simulink model "six_dof_COMPUTED_TORQUE"  (R2021b)
settings: Solver=ode4  StartTime=0.0  StopTime=10.0  FixedStep=1/100  RelTol=1e-3
libraries: robotmaniplib x4, simulink x2
settings Model: Creator=HP  LastModifiedBy=marco

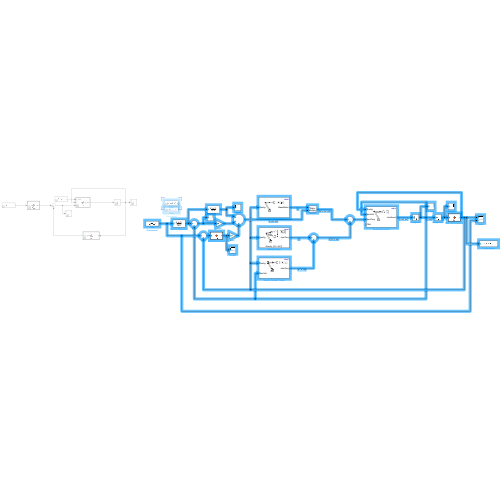
[thumbnail: Simulink's stored preview of the top-level diagram]
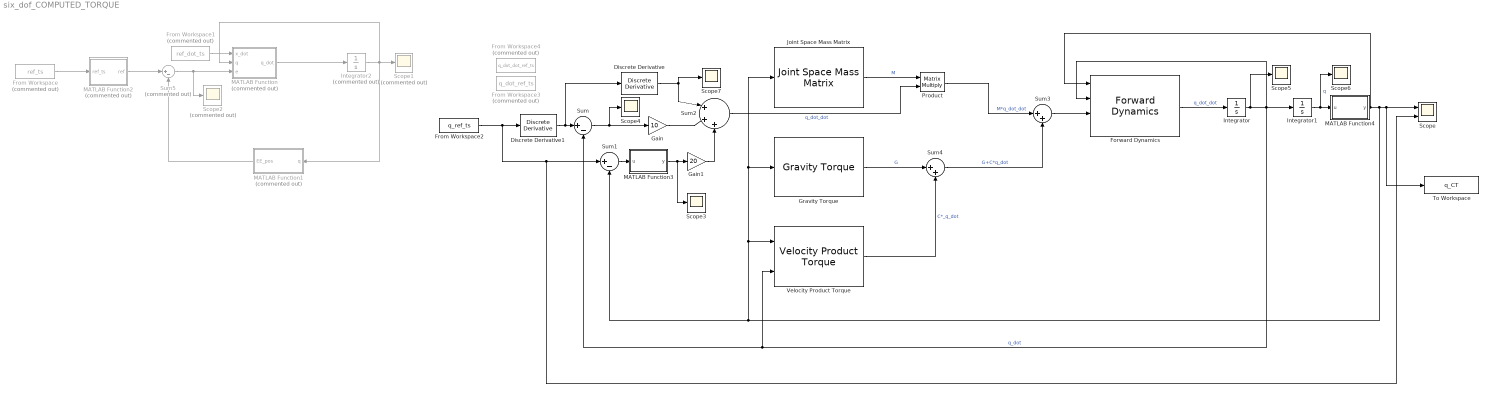
== system six_dof_COMPUTED_TORQUE ==
  Discrete Derivative : simulink/Discrete/Discrete Derivative  gainval=1.0  ICPrevScaledInput=0.0  OutMin=[]  OutMax=[]  OutDataType=fixdt(1, 16)  OutScaling=2^-10  DoSatur=off
  Discrete Derivative1 : simulink/Discrete/Discrete Derivative  gainval=1.0  ICPrevScaledInput=0.0  OutMin=[]  OutMax=[]  OutDataType=fixdt(1, 16)  OutScaling=2^-10  DoSatur=off
  Forward Dynamics : robotmaniplib/Forward Dynamics  RigidBodyTree=robot  SimulateUsing=Interpreted execution
  From Workspace : FromWorkspace  Commented=on  VariableName=ref_ts
  From Workspace1 : FromWorkspace  Commented=on  VariableName=ref_dot_ts
  From Workspace2 : FromWorkspace  VariableName=q_ref_ts
  From Workspace3 : FromWorkspace  Commented=on  VariableName=q_dot_ref_ts
  From Workspace4 : FromWorkspace  Commented=on  VariableName=q_dot_dot_ref_ts
  Gain : Gain  Gain=10
  Gain1 : Gain  Gain=20
  Gravity Torque : robotmaniplib/Gravity Torque  RigidBodyTree=robot  SimulateUsing=Interpreted execution
  Integrator : Integrator  InitialCondition=[0; 0; 0; 0; 0; 0]  LimitOutput=on  UpperSaturationLimit=[pi/2; pi/2; pi/2; pi/2; pi/2; pi/2]  LowerSaturationLimit=-[pi/2; pi/2; pi/2; pi/2; pi/2; pi/2]
  Integrator1 : Integrator  InitialCondition=[0; 0; 0; 0; pi/2; 0]  LimitOutput=on  UpperSaturationLimit=[pi; pi/4; 5*pi/4; pi; 5*pi/4; pi]  LowerSaturationLimit=-[pi; 5*pi/4; pi/4; pi; 5*pi/4; pi]
  Integrator2 : Integrator  Commented=on
  Joint Space Mass Matrix : robotmaniplib/Joint Space Mass Matrix  RigidBodyTree=robot  SimulateUsing=Interpreted execution
  MATLAB Function : MATLAB Function  Commented=on  TreatAsAtomicUnit=on
  MATLAB Function1 : MATLAB Function  Commented=on  TreatAsAtomicUnit=on
  MATLAB Function2 : MATLAB Function  Commented=on  TreatAsAtomicUnit=on
  MATLAB Function3 : MATLAB Function  TreatAsAtomicUnit=on
  MATLAB Function4 : MATLAB Function  TreatAsAtomicUnit=on
  Product : Product  Multiplication=Matrix(*)
  Scope : Scope  NumInputPorts=2
  Scope1 : Scope  Commented=on
  Scope2 : Scope  Commented=on
  Scope{3..7} (5 alike) : Scope
  Sum : Sum  Inputs=|+-
  Sum1 : Sum  Inputs=|+-
  Sum2 : Sum  Inputs=|+++
  Sum3 : Sum  Inputs=|++
  Sum4 : Sum  Inputs=|++
  Sum5 : Sum  Commented=on  Inputs=|+-
  To Workspace : ToWorkspace  VariableName=q_CT  SaveFormat=Timeseries  SampleTime=-1
  Velocity Product Torque : robotmaniplib/Velocity Product Torque  RigidBodyTree=robot  SimulateUsing=Interpreted execution
      settings: SourceProductBaseCode=RO
  wires:
  Sum/1 -> Scope4/1, Gain/1
  Sum1/1 -> MATLAB Function3/1(u)
  Joint Space Mass Matrix/1 -> Product/1  "M"
  Gain/1 -> Sum2/2
  Gain1/1 -> Sum2/3
  Sum2/1 -> Product/2  "q_dot_dot"
  Sum3/1 -> Forward Dynamics/3
  Gravity Torque/1 -> Sum4/1  "G"
  Velocity Product Torque/1 -> Sum4/2  "C*_q_dot"
  Product/1 -> Sum3/1  "M*q_dot_dot"
  Sum4/1 -> Sum3/2  "G+C*q_dot"
  Forward Dynamics/1 -> Integrator/1  "q_dot_dot"
  Integrator/1 -> Scope5/1, Velocity Product Torque/2, Sum/2, Forward Dynamics/2, Integrator1/1  "q_dot"
  Integrator1/1 -> Scope6/1, MATLAB Function4/1(u)  "q"
  From Workspace/1 -> MATLAB Function2/1(ref_ts)
  MATLAB Function/1(q_dot) -> Integrator2/1
  Sum5/1 -> Scope2/1, MATLAB Function/3(e)
  Integrator2/1 -> MATLAB Function/2(q), Scope1/1, MATLAB Function1/1(q)
  MATLAB Function1/1(EE_pos) -> Sum5/2
  From Workspace1/1 -> MATLAB Function/1(x_dot)
  MATLAB Function2/1(ref) -> Sum5/1
  From Workspace2/1 -> Discrete Derivative1/1, Scope/2, Sum1/1
  MATLAB Function3/1(y) -> Scope3/1, Gain1/1
  MATLAB Function4/1(y) -> Velocity Product Torque/1, Joint Space Mass Matrix/1, Gravity Torque/1, Sum1/2, To Workspace/1, Scope/1, Forward Dynamics/1
  Discrete Derivative/1 -> Scope7/1, Sum2/1
  Discrete Derivative1/1 -> Discrete Derivative/1, Sum/1

== matlab function six_dof_COMPUTED_TORQUE/MATLAB Function ==
  data: x_dot input; q_dot output; q input; e input
function q_dot = fcn(x_dot, q, e)
    q1 = q(1);
    q2 = q(2);
    q3 = q(3);
    q4 = q(4);
    q5 = q(5);
    q6 = q(6);
J_a_now = eval(J_a);
K = blkdiag(100*eye(3),30*eye(3));
q_dot = J_a_now\(x_dot'+K*e);

== matlab function six_dof_COMPUTED_TORQUE/MATLAB Function2 ==
  data: ref_ts input; ref output
function ref = fcn(ref_ts)

ref = ref_ts';

== matlab function six_dof_COMPUTED_TORQUE/MATLAB Function3 ==
  data: u input; y output
function y = fcn(u)

y = wrapToPi(u);

== matlab function six_dof_COMPUTED_TORQUE/MATLAB Function4 ==
  data: u input; y output
function y = fcn(u)

y = wrapToPi(u);

== matlab function six_dof_COMPUTED_TORQUE/MATLAB Function1 ==
  data: q input; EE_pos output
function EE_pos = fcn(q)
poseNow = getTransform(robot,q(:),'L6');
angle_now = rotm2eul(poseNow(1:3, 1:3)); 
EE_pos = [poseNow(1,4); poseNow(2,4); poseNow(3,4); angle_now'];
